simulink model "first_example_in_class"  (R2023a)
settings: Solver=VariableStepAuto  StartTime=0.0  StopTime=10.0  RelTol=1e-3
undefined symbols (not defined in the file or in its folder): degConv
settings Model: Creator=Administrator  LastModifiedBy=Administrator

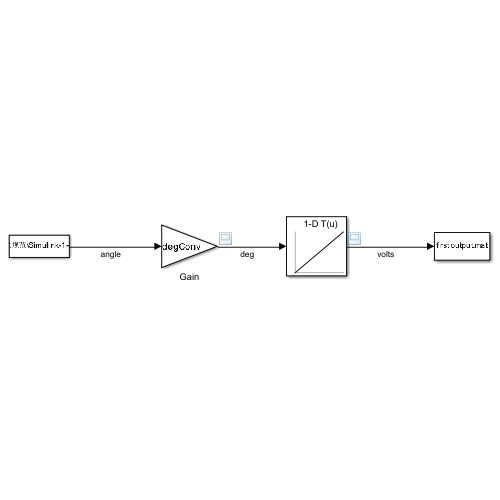
[thumbnail: Simulink's stored preview of the top-level diagram]
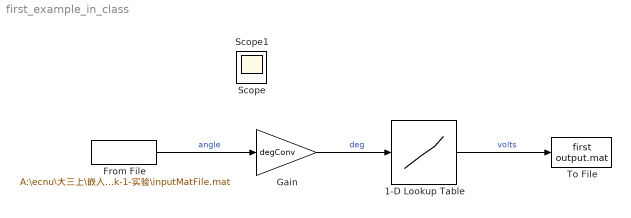
== system first_example_in_class ==
  1-D Lookup Table : Lookup_n-D  NumberOfTableDimensions=1  BreakpointsForDimension1=[0 90]  Table=[0.5 4.5]  InternalRulePriority=Speed  RndMeth=Simplest
  From File : FromFile  FileName=A:\ecnu\大三上\嵌入式规范\Simulink-1-实验\inputMatFile.mat  SampleTime=0
  Gain : Gain  Gain=degConv
  To File : ToFile  Filename=first output.mat  SaveFormat=Timeseries
  Scope : Scope
  Scope1 : Scope
  wires:
  Gain/1 -> 1-D Lookup Table/1  "deg"
  From File/1 -> Gain/1  "angle"
  1-D Lookup Table/1 -> To File/1  "volts"
